simulink model "task"  (R2024b)
settings: Solver=FixedStepAuto  StartTime=0.0  StopTime=50  FixedStep=0.01  RelTol=1e-3
libraries: simulink x1
settings Model: Creator=ryoga  LastModifiedBy=ryoga

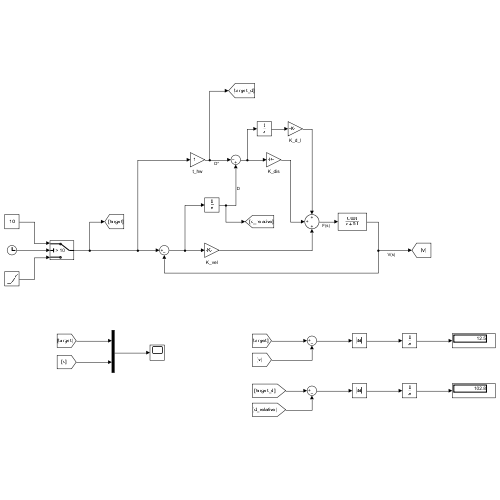
[thumbnail: Simulink's stored preview of the top-level diagram]
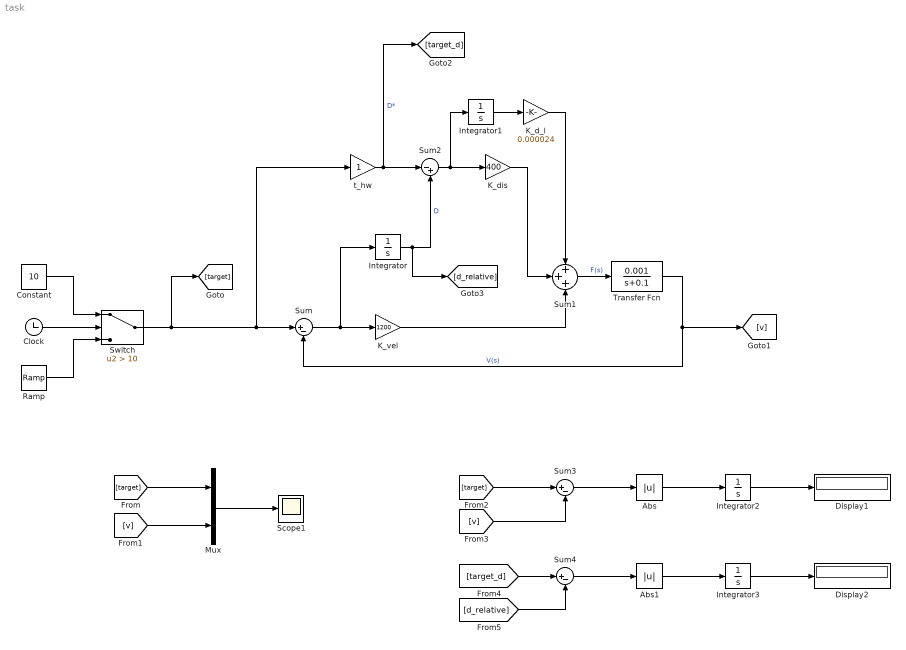
== system task ==
  Abs : Abs  SaturateOnIntegerOverflow=off
  Abs1 : Abs  SaturateOnIntegerOverflow=off
  Clock : Clock
  Constant : Constant  Value=10
  Display1 : Display
  Display2 : Display
  Integrator{,1..3} (4 alike) : Integrator
  K_d_l : Gain  Gain=0.000024
  K_dis : Gain  Gain=400
  K_vel : Gain  Gain=1200
  Mux : Mux  Inputs=2
  Ramp : simulink/Sources/Ramp  slope=1  start=0  InitialOutput=0
  Scope1 : Scope
  Sum : Sum  Inputs=|+-
  Sum1 : Sum  Inputs=+++
  Sum2 : Sum  Inputs=|-+
  Sum3 : Sum  Inputs=|+-
  Sum4 : Sum  Inputs=|+-
  Switch : Switch  Criteria=u2 > Threshold  Threshold=10  SaturateOnIntegerOverflow=off  InputSameDT=off
  Transfer Fcn : TransferFcn  Numerator=[0.001]  Denominator=[1 0.1]
  t_hw : Gain
  wires:
  Sum1/1 -> Transfer Fcn/1  "F(s)"
  Transfer Fcn/1 -> [v], Sum/2  "V(s)"
  K_vel/1 -> Sum1/3
  Sum/1 -> Integrator/1, K_vel/1
  Integrator/1 -> [d_relative], Sum2/2  "D"
  Sum2/1 -> Integrator1/1, K_dis/1
  Integrator1/1 -> K_d_l/1
  K_dis/1 -> Sum1/2
  K_d_l/1 -> Sum1/1
  t_hw/1 -> [target_d], Sum2/1  "D*"
  Constant/1 -> Switch/1
  Clock/1 -> Switch/2
  Ramp/1 -> Switch/3
  Switch/1 -> [target], t_hw/1, Sum/1
  [target] -> Mux/1
  Mux/1 -> Scope1/1
  [v] -> Mux/2
  [target] -> Sum3/1
  [v] -> Sum3/2
  Sum3/1 -> Abs/1
  Abs/1 -> Integrator2/1
  Integrator2/1 -> Display1/1
  [d_relative] -> Sum4/2
  [target_d] -> Sum4/1
  Integrator3/1 -> Display2/1
  Abs1/1 -> Integrator3/1
  Sum4/1 -> Abs1/1
